simulink model "CS_esquema"  (R2013a)
settings: Solver=FixedStepDiscrete  StartTime=0.0  StopTime=5  FixedStep=0.1  RelTol=1e-3
StopFcn:
  | salida(aux1,aux2,aux3,man)
undefined symbols (not defined in the file or in its folder): A, B, DiscIntNeverNeededParam, Humusoft, MF624
libraries: rtwinlib x3
settings Model: SimulationMode=external  ExtModeTrigDuration=10000  Creator=Equipo-Servo  LastModifiedBy=Equipo-Servo
settings HardwareCC: ProdIntDivRoundTo=Zero  ProdEndianess=LittleEndian  ProdHWDeviceType=Generic->32-bit x86 compatible
settings RTWCC: SystemTargetFile=rtwin.tlc  TemplateMakefile=rtwin.tmf  Description=Real-Time Windows Target  ProcessScript=rtwin_make_rtw_hook  RTWCompilerOptimization=On
settings CodeAppCC: MaxIdLength=95
settings RTWinTargetCC: TargetLibSuffix=_rtwin.lib  TargetPreCompLibLocation=C:\Program Files\MATLAB\R2013a\toolbox\rtw\targets\rtwin\lib\win32  CodeReplacementLibrary=ANSI_C  RTWinDir=C:/PROGRA~1/MATLAB/R2013a/toolbox/rtw/targets/rtwin  TargetArch=win32

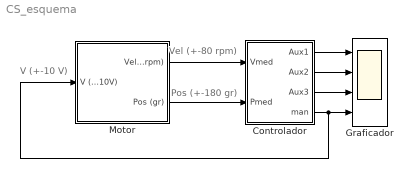
== system CS_esquema ==
  note: Vel (+-80 rpm)
  note: Pos (+-180 gr)
  note: V (+-10 V)
  Controlador : Subsystem
  Graficador : Scope  NumInputPorts=4
      settings: TimeRange=5  YMin=-50~-100~-50~-10  YMax=50~100~50~10  SampleTime=Tm
  Motor : Subsystem
  wires:
  Controlador/4(man) -> Motor/1(V (+-10V)), Graficador/4
  Motor/1(Vel (rpm)) -> Controlador/1(Vmed)
  Motor/2(Pos (gr)) -> Controlador/2(Pmed)
  Controlador/1(Aux1) -> Graficador/1
  Controlador/3(Aux3) -> Graficador/3
  Controlador/2(Aux2) -> Graficador/2

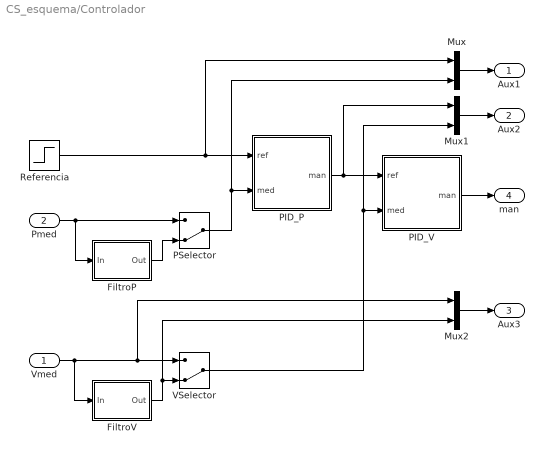
== system CS_esquema/Controlador ==
  Vmed : Inport
  Pmed : Inport  Port=2
  FiltroP : Subsystem  mask{N=2, Fc=1, Fm=1/0.1}
      mask prompts: N "Orden del filtro (Butterworth)"; Fc "Frecuencia de corte (Fc<Fm/2)"; Fm "Frecuencia de muestreo"
      mask init:
      | Fn = Fm/2;   % Frecuencia de Nyquist
      | [B,A] = butter(N,Fc/Fn);
  FiltroV : Subsystem  mask{N=2, Fc=1, Fm=1/0.1}
      mask prompts: N "Orden del filtro (Butterworth)"; Fc "Frecuencia de corte (Fc<Fm/2)"; Fm "Frecuencia de muestreo"
      mask init:
      | Fn = Fm/2;   % Frecuencia de Nyquist
      | [B,A] = butter(N,Fc/Fn);
  Mux : Mux  Inputs=2
  Mux1 : Mux  Inputs=2
  Mux2 : Mux  Inputs=2
  PID_P : Subsystem  mask{P=1, I=0, D=0, Tm=0.1, Kb=1, Fc=5, Mmx=80, Mmn=-80}
      mask prompts: P "Ganancia Proporcional"; I "Ganancia Integral"; D "Ganancia Derivativa"; Tm "Período de muestreo"; Kb "Ganancia Antiwindup"; Fc "Fc Filtro D"; Mmx "Mando máximo"; Mmn "Mando mínimo"
      mask init:
      | N=2*pi*Fc;
  PID_V : Subsystem  mask{P=1, I=0, D=0, Tm=0.1, Kb=1, Fc=5, Mmx=10, Mmn=-10}
      mask prompts: P "Ganancia Proporcional"; I "Ganancia Integral"; D "Ganancia Derivativa"; Tm "Período de muestreo"; Kb "Ganancia Antiwindup"; Fc "Fc Filtro D"; Mmx "Mando máximo"; Mmn "Mando mínimo"
      mask init:
      | N=2*pi*Fc;
  PSelector : ManualSwitch  CurrentSetting=0
  Referencia : Step  Time=2  Before=-50  After=50  SampleTime=0
  VSelector : ManualSwitch  CurrentSetting=0
  Aux1 : Outport
  Aux2 : Outport  Port=2
  Aux3 : Outport  Port=3
  man : Outport  Port=4
  wires:
  Mux2/1 -> Aux3/1
  Mux1/1 -> Aux2/1
  Mux/1 -> Aux1/1
  PSelector/1 -> Mux/2, PID_P/2(med)
  FiltroP/1(Out) -> PSelector/2
  VSelector/1 -> Mux1/2, PID_V/2(med)
  FiltroV/1(Out) -> VSelector/2, Mux2/2
  Vmed/1 -> VSelector/1, Mux2/1, FiltroV/1(In)
  PID_V/1(man) -> man/1
  PID_P/1(man) -> Mux1/1, PID_V/1(ref)
  Pmed/1 -> PSelector/1, FiltroP/1(In)
  Referencia/1 -> PID_P/1(ref), Mux/1

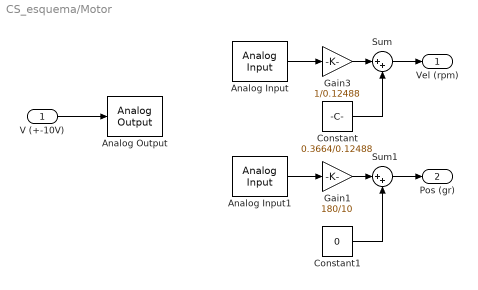
== system CS_esquema/Motor ==
  V (+-10V) : Inport
  Analog Input : rtwinlib/Analog Input  SampleTime=-1  MaxMissedTicks=10  ShowMissedTicks=off  YieldWhenWaiting=off  DrvName=Humusoft/MF624  DrvAddress=0  DrvOptions=0  Channels=1  RangeMode=1  VoltRange=1  DataType=1
      settings: AttributesFormatString=Humusoft\nMF624 [0h]
  Analog Input1 : rtwinlib/Analog Input  SampleTime=-1  MaxMissedTicks=10  ShowMissedTicks=off  YieldWhenWaiting=off  DrvName=Humusoft/MF624  DrvAddress=0  DrvOptions=0  Channels=2  RangeMode=1  VoltRange=1  DataType=1
      settings: AttributesFormatString=Humusoft\nMF624 [0h]
  Analog Output : rtwinlib/Analog Output  SampleTime=-1  MaxMissedTicks=10  ShowMissedTicks=off  YieldWhenWaiting=off  DrvName=Humusoft/MF624  DrvAddress=0  DrvOptions=0  Channels=1  RangeMode=1  VoltRange=1  InitialValue=0  FinalValue=0
      settings: AttributesFormatString=Humusoft\nMF624 [0h]
  Constant : Constant  Value=0.3664/0.12488
  Constant1 : Constant  Value=0
  Gain1 : Gain  Gain=180/10
  Gain3 : Gain  Gain=1/0.12488
  Sum : Sum  Inputs=|++
  Sum1 : Sum  Inputs=|++
  Vel (rpm) : Outport
  Pos (gr) : Outport  Port=2
  wires:
  V (+-10V)/1 -> Analog Output/1
  Analog Input/1 -> Gain3/1
  Constant/1 -> Sum/2
  Sum/1 -> Vel (rpm)/1
  Gain3/1 -> Sum/1
  Analog Input1/1 -> Gain1/1
  Constant1/1 -> Sum1/2
  Gain1/1 -> Sum1/1
  Sum1/1 -> Pos (gr)/1

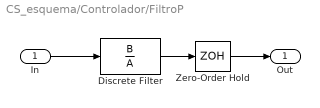
== system CS_esquema/Controlador/FiltroP ==
  In : Inport
  Discrete Filter : DiscreteFilter  Numerator=B  Denominator=A  SampleTime=1/Fm
  Zero-Order Hold : ZeroOrderHold  SampleTime=1/Fm
  Out : Outport
  wires:
  Zero-Order Hold/1 -> Out/1
  In/1 -> Discrete Filter/1
  Discrete Filter/1 -> Zero-Order Hold/1

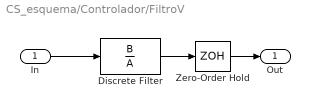
== system CS_esquema/Controlador/FiltroV ==
  In : Inport
  Discrete Filter : DiscreteFilter  Numerator=B  Denominator=A  SampleTime=1/Fm
  Zero-Order Hold : ZeroOrderHold  SampleTime=1/Fm
  Out : Outport
  wires:
  Zero-Order Hold/1 -> Out/1
  Discrete Filter/1 -> Zero-Order Hold/1
  In/1 -> Discrete Filter/1

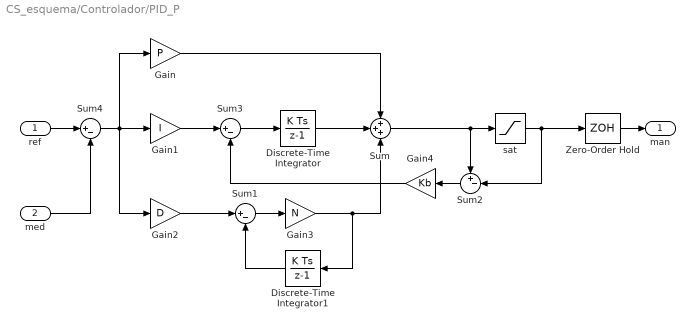
== system CS_esquema/Controlador/PID_P ==
  ref : Inport
  med : Inport  Port=2
  Discrete-Time Integrator : DiscreteIntegrator  SampleTime=Tm  ICPrevOutput=DiscIntNeverNeededParam  ICPrevScaledInput=DiscIntNeverNeededParam
  Discrete-Time Integrator1 : DiscreteIntegrator  SampleTime=Tm  ICPrevOutput=DiscIntNeverNeededParam  ICPrevScaledInput=DiscIntNeverNeededParam
  Gain : Gain  Gain=P
  Gain1 : Gain  Gain=I
  Gain2 : Gain  Gain=D
  Gain3 : Gain  Gain=N
  Gain4 : Gain  Gain=Kb
  Sum : Sum  Inputs=+++
  Sum1 : Sum  Inputs=|+-
  Sum2 : Sum  Inputs=+-|
  Sum3 : Sum  Inputs=|+-
  Sum4 : Sum  Inputs=|+-
  Zero-Order Hold : ZeroOrderHold  SampleTime=Tm
  sat : Saturate  UpperLimit=Mmx  LowerLimit=Mmn
  man : Outport
  wires:
  Zero-Order Hold/1 -> man/1
  ref/1 -> Sum4/1
  med/1 -> Sum4/2
  Gain1/1 -> Sum3/1
  sat/1 -> Zero-Order Hold/1, Sum2/2
  Sum/1 -> sat/1, Sum2/1
  Sum2/1 -> Gain4/1
  Discrete-Time Integrator/1 -> Sum/2
  Sum1/1 -> Gain3/1
  Gain4/1 -> Sum3/2
  Gain/1 -> Sum/1
  Gain3/1 -> Discrete-Time Integrator1/1, Sum/3
  Sum4/1 -> Gain1/1, Gain/1, Gain2/1
  Sum3/1 -> Discrete-Time Integrator/1
  Discrete-Time Integrator1/1 -> Sum1/2
  Gain2/1 -> Sum1/1

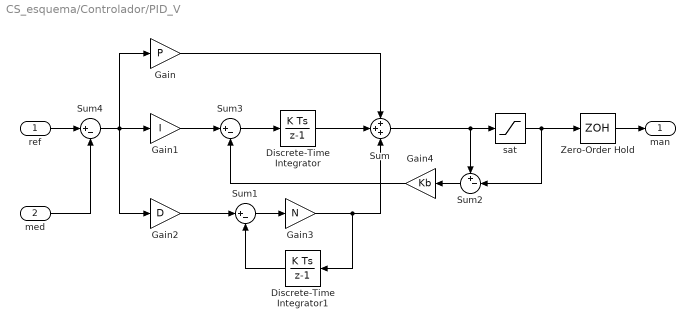
== system CS_esquema/Controlador/PID_V ==
  ref : Inport
  med : Inport  Port=2
  Discrete-Time Integrator : DiscreteIntegrator  SampleTime=Tm  ICPrevOutput=DiscIntNeverNeededParam  ICPrevScaledInput=DiscIntNeverNeededParam
  Discrete-Time Integrator1 : DiscreteIntegrator  SampleTime=Tm  ICPrevOutput=DiscIntNeverNeededParam  ICPrevScaledInput=DiscIntNeverNeededParam
  Gain : Gain  Gain=P
  Gain1 : Gain  Gain=I
  Gain2 : Gain  Gain=D
  Gain3 : Gain  Gain=N
  Gain4 : Gain  Gain=Kb
  Sum : Sum  Inputs=+++
  Sum1 : Sum  Inputs=|+-
  Sum2 : Sum  Inputs=+-|
  Sum3 : Sum  Inputs=|+-
  Sum4 : Sum  Inputs=|+-
  Zero-Order Hold : ZeroOrderHold  SampleTime=Tm
  sat : Saturate  UpperLimit=Mmx  LowerLimit=Mmn
  man : Outport
  wires:
  Zero-Order Hold/1 -> man/1
  Gain2/1 -> Sum1/1
  Discrete-Time Integrator1/1 -> Sum1/2
  Sum3/1 -> Discrete-Time Integrator/1
  Sum4/1 -> Gain2/1, Gain/1, Gain1/1
  Gain3/1 -> Sum/3, Discrete-Time Integrator1/1
  Gain/1 -> Sum/1
  Gain4/1 -> Sum3/2
  Sum1/1 -> Gain3/1
  Discrete-Time Integrator/1 -> Sum/2
  Sum2/1 -> Gain4/1
  Sum/1 -> Sum2/1, sat/1
  sat/1 -> Sum2/2, Zero-Order Hold/1
  Gain1/1 -> Sum3/1
  med/1 -> Sum4/2
  ref/1 -> Sum4/1
